simulink model "UART_test"  (R2020a)
settings: Solver=FixedStepAuto  StartTime=0.0  StopTime=10.0  FixedStep=1e-3  RelTol=1e-3  EnableMultiTasking=on
libraries: etargetslib x17, frdmk64flib x10, simulink x1
(part 3 of 3)

== stateflow chart UART_test/DCM Communication Subsystem/Communication from DCM Subsystem/Communication Out Switcher ==
  note: Communication out Switcher:
      | % help switch between echo and egram communication modes
      | 	if ECHO_SWITCH is true:
      | 		send only 1 programmable-parameters package
      | 	If EGRAM_SWITCH is true:
      | 		send a egram data package once per 1ms by switching COMM_OUT_SWITCH between 0/1
  state egram_stop
    % egram low stage
    % wait for 1ms to send next egram package
    entry:
    COMM_OUT_SWITCH=0;
  state comm_stop
    % stop communication
    entry:
    COMM_OUT_SWITCH=0;
  state egram_pulse
    % egram high stage (pulse)
    % send a egram data package
    entry:
    COMM_OUT_SWITCH=2;
  state echo_s_pulse
    % send a programmable-parameters package
    % 1ms delay allows enough time for DCM to read
    entry:
    COMM_OUT_SWITCH=1;
  (default) -> comm_stop
  egram_stop -> comm_stop [order 2] : [ECHO_SWITCH==true]
  comm_stop -> egram_stop [order 2] : [EGRAM_SWITCH==true]
  comm_stop -> echo_s_pulse [order 1] : [ECHO_SWITCH==true]
  echo_s_pulse -> comm_stop
  egram_pulse -> comm_stop [order 1] : [EGRAM_SWITCH==false | ECHO_SWITCH==true]
  egram_pulse -> egram_stop [order 2]
  egram_stop -> egram_pulse [order 1] : [after(100,msec)]
  data: EGRAM_SWITCH input boolean; COMM_OUT_SWITCH output uint8; ECHO_SWITCH input boolean

== stateflow chart UART_test/DCM Communication Subsystem/Communication from DCM Subsystem/UART Interpretation ==
  settings: executeAtInitialization=1
  note: UART Interpretation Chart:
      | This chart interprets data received from DCM communication.
      | There’re four types of package pacemaker can receive: set_r, echo_r, egram_r, and stopegram_r. (Documentation section 3.3.2)
      | After a package of 59 bytes is received, status==0, then operate the following 4 steps:
      | 1. Validate Sync byte. If not valid, ignore this package and wait for next package.
      | 2. Validate Checksum. If not valid, ignore this package and wait for next package.
      | 3. Operate according to FnCode (set_r, echo_r, egram_r, or stopegram_r).
      | 4. Wait for next package.
      | Inputs:
      | data and status from UART0 block
      | Outpus:
      | 1. DCM_Inputbus data
      | 2. EGRAM_SWITCH and ECHO_SWITCH: tell pacemaker to send egram/pparams data back to DCM
      | 3. PPARAM_UPDATE: tell pacemaker if new set of programmable parameters are received, so that pacing modes should be updated
      |
      | Note:
      | The matlab function bitsxor() is used to calculate checksum of data received.
  state set_r
    entry:
    % store parameters values from DCM
    MODE = data(3);
    LRL = data(4);
    URL = data(5);
    MAX_SENSOR_RATE = data(6);
    AV_DELAY_FIXED = typecast(data(7: 8), 'uint16');
    AV_DELAY_DYNAMIC = data(9);
    MIN_AV_DELAY_DYNAMIC = data(10);
    AV_DELAY_OFFSET_SENSED =  typecast(data(11), 'int8');
    ATR_AMP_REG = typecast(data(12: 15), 'single');
    VENT_AMP_REG = typecast(data(16: 19), 'single');
    ATR_AMP_UNREG = typecast(data(20: 23), 'single');
    VENT_AMP_UNREG = typecast(data(24: 27), 'single');
    ATR_PULSE_WIDTH = data(28);
    VENT_PULSE_WIDTH = data(29);
    ATR_SENSITIVITY = typecast(data(30: 33), 'single');
    VENT_SENSITIVITY = typecast(data(34: 37), 'single');
    VRP = typecast(data(38: 39), 'uint16');
    ARP = typecast(data(40: 41), 'uint16');
    PVARP = typecast(data(42: 43), 'uint16');
    PVARP_EXT = typecast(data(44: 45), 'uint16');
    HYSTERESIS_LIMIT = data(46);
    RATE_SMOOTHING = data(47);
    ATR_MODE = data(48);
    ATR_DURATION = typecast(data(49: 50), 'uint16');
    ATR_FALLBACK_TIME = typecast(data(51: 52), 'uint16');
    VENT_BLANKING = data(53);
    ACT_THRESHOLD = data(54);
    REACTION_TIME = data(55);
    RESPONSE_FACTOR = data(56);
    RECOVERY_TIME = typecast(data(57: 58), 'uint16');
    B_LED=true;
    % package received signal
    PPARAM_UPDATE=true;
  note: % Disable Activity Sensing Subsystem if not in Rate Adaptive Pacing Mode
  state Init
    entry:
    % parameters have default values if no data received
    MODE=15; % change to DDD in the future
    LRL = 60;
    URL = 120;
    MAX_SENSOR_RATE = 120;
    AV_DELAY_FIXED = 150;
    AV_DELAY_DYNAMIC = 0;
    MIN_AV_DELAY_DYNAMIC = 50;
    AV_DELAY_OFFSET_SENSED = 0;
    ATR_AMP_REG = 5;
    VENT_AMP_REG = 5;
    ATR_AMP_UNREG = 3.75;
    VENT_AMP_UNREG = 3.75;
    ATR_PULSE_WIDTH = 1;
    VENT_PULSE_WIDTH = 1;
    ATR_SENSITIVITY = 4;
    VENT_SENSITIVITY = 4;
    VRP = 320;
    ARP = 250;
    PVARP = 250;
    PVARP_EXT = 0;
    HYSTERESIS_LIMIT = 0;
    RATE_SMOOTHING = 0;
    ATR_MODE = 0;
    ATR_DURATION = 20;
    ATR_FALLBACK_TIME = 60;
    VENT_BLANKING = 40;
    ACT_THRESHOLD = 3; %3
    REACTION_TIME = 3; %30
    RESPONSE_FACTOR = 16; %8
    RECOVERY_TIME = 3; %300
    % local variables that turn egram/echo communication out modules on/off
    EGRAM_SWITCH=false;
    ECHO_SWITCH=false;
    % signal that represents if programmable parameters are received
    PPARAM_UPDATE=false;
    % turn Activity Sensing Subsystem on/off
    ACT_SENSING_SWITCH=true; %false
  state echo_r
    % send a parameter package to DCM
    entry:
    ECHO_SWITCH=true;
    G_LED=true;
  state Checksum
    entry:
    % compare checksum first
    % if checksum is valid, operate according to FnCode
    CHECKSUM=data(59);
    CHECKSUM_REAL=bitsxor(data(1:58));
    B_LED=false;
    G_LED=false;
  state Standby
    %Waiting for Data
    exit:
    % rxdata must be stored initially, otherwise rxdata
    % changes after Checksum. The reason is rxdata
    % reset to zeros after all data have been read
    data=rxdata;
  state stopegram_r
    % stop sending egram to DCM
    entry:
    EGRAM_SWITCH=false;
    R_LED=false;
  state egram_r
    % start sending a egram package
    % to DCM every 1ms
    entry:
    EGRAM_SWITCH=true;
    R_LED=true;
  (junction 95) -> Standby [order 1] : [MODE==11 || MODE==12 || MODE==13 || MODE==14 || MODE==15 || MODE==16 || MODE==17 || MODE==18]{ACT_SENSING_SWITCH=true}
  set_r -> (junction 95) : {PPARAM_UPDATE=false}
  (junction 95) -> Standby [order 2] : {ACT_SENSING_SWITCH=false}
  (default) -> Init
  (junction 45) -> set_r [order 1] : [data(2)==0x00]
  echo_r -> Standby : {ECHO_SWITCH=false}
  (junction 45) -> Standby [order 5]
  (junction 45) -> echo_r [order 2] : [data(2)==0x01]
  Checksum -> Standby [order 2]
  (junction 41) -> Standby [order 2]
  Checksum -> (junction 45) [order 1] : [CHECKSUM_REAL==CHECKSUM]
  (junction 45) -> egram_r [order 3] : [data(2)==0x02]
  (junction 45) -> stopegram_r [order 4] : [data(2)==0x03]
  Init -> Standby
  Standby -> (junction 41) : [status==0]
  (junction 41) -> Checksum [order 1] : [rxdata(1)==0x55]
  egram_r -> Standby
  stopegram_r -> Standby
  data: checksum function_output uint8 size=1; data_array function_input uint8; MODE output uint8; LRL output uint8; URL output uint8; MAX_SENSOR_RATE output uint8; AV_DELAY_FIXED output uint16; AV_DELAY_DYNAMIC output uint8; MIN_AV_DELAY_DYNAMIC output uint8; AV_DELAY_OFFSET_SENSED output int8; ATR_AMP_REG output single; VENT_AMP_REG output single; ATR_AMP_UNREG output single; VENT_AMP_UNREG output single; ATR_PULSE_WIDTH output uint8; VENT_PULSE_WIDTH output uint8; ATR_SENSITIVITY output single; VENT_SENSITIVITY output single; VRP output uint16; ARP output uint16; PVARP output uint16; PVARP_EXT output uint16; HYSTERESIS_LIMIT output uint8; RATE_SMOOTHING output uint8; ATR_MODE output uint8; ATR_DURATION output uint16; ATR_FALLBACK_TIME output uint16; VENT_BLANKING output uint8; rxdata input uint8; status input uint8; ACT_THRESHOLD output uint8; REACTION_TIME output uint8; RESPONSE_FACTOR output uint8; RECOVERY_TIME output uint16; CHECKSUM_REAL local uint8 size=1; CHECKSUM local uint8 size=1; EGRAM_SWITCH output boolean; ECHO_SWITCH output boolean; data local uint8; PPARAM_UPDATE output boolean; ACT_SENSING_SWITCH output boolean; B_LED output boolean; G_LED output boolean; R_LED output boolean
  function checksum=bitsxor(data_array):
    | function checksum=bitsxor(data_array)
    |     % calculate checksum
    |     % input: data_array is array of uint8 numbers
    |     % output: checksum (uint8) is bit-wise XOR of all uint8 data in the array
    |     checksum=data_array(1);
    |     for i=2:length(data_array)
    |         checksum = bitxor(checksum,data_array(i)); 
    |     end
    | end
